simulink model "arduino_smart_plant1"  (R2024a)
settings: Solver=FixedStepAuto  StartTime=0.0  StopTime=30  RelTol=1e-3  EnableMultiTasking=on
undefined symbols (not defined in the file): Fi, Wi
libraries: arduinolib x5, arduinowifilib x4
settings Model: ExtModeTrigDuration=2  Creator=The MathWorks, Inc.  LastModifiedBy=josep
settings SolverCC: AlgebraicLoopSolver=TrustRegion
settings DataIOCC: ReturnWorkspaceOutputs=off
settings OptimizationCC: MaxStackSize=64
settings DebuggingCC: ParameterTunabilityLossMsg=error  UnconnectedInputMsg=warning  UnconnectedOutputMsg=warning  UnconnectedLineMsg=warning  ArithmeticOperatorsInVariantConditions=warning
settings HardwareCC: ProdBitPerInt=16  ProdBitPerPointer=16  ProdBitPerSizeT=16  ProdBitPerPtrDiffT=16  ProdLargestAtomicFloat=None  ProdWordSize=8  ProdHWDeviceType=Atmel->AVR  UseEmbeddedCoderFeatures=off  UseSimulinkCoderFeatures=off
settings ModelReferenceCC: EnableRefExpFcnMdlSchedulingChecks=on
settings SFSimCC: SimUseLocalCustomCode=off
settings RTWCC: Description=Embedded Coder  SystemTargetFile=ert.tlc  HardwareBoard=Arduino Mega 2560  TemplateMakefile=ert_default_tmf  GenerateReport=on  RTWUseLocalCustomCode=off  Toolchain=Arduino AVR  BuildConfiguration=Faster Runs  LaunchReport=on  GPUComputeCapability=3.5
settings CodeAppCC: ForceParamTrailComments=on  OperatorAnnotations=on  StateflowObjectComments=on  MATLABSourceComments=on
settings ERTTargetCC: ERTCustomFileBanners=off  SupportContinuousTime=on  SupportNonInlinedSFcns=on  RemoveResetFunc=off  SupportVariableSizeSignals=on  ModelStepFunctionPrototypeControlCompliant=off

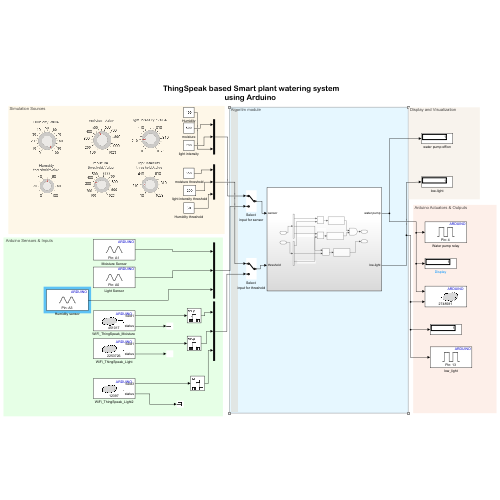
[thumbnail: Simulink's stored preview of the top-level diagram]
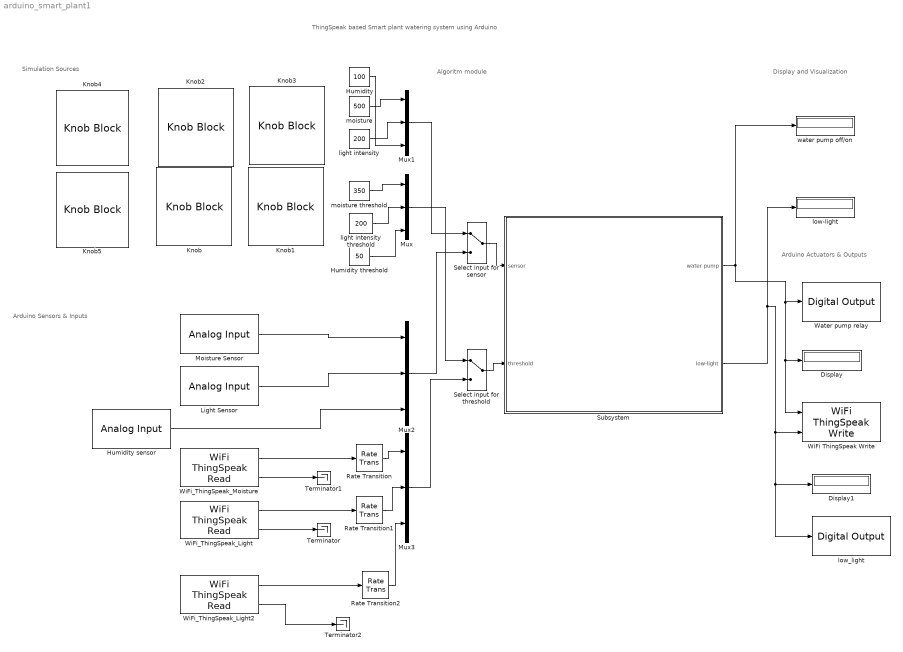
== system arduino_smart_plant1 ==
  note: Display and Visualization
  note: ThingSpeak based Smart plant watering system
      | using Arduino
  note: Simulation Sources
  note: Algoritm module
  note: Arduino Sensors & Inputs
  note: Arduino Actuators & Outputs
  " moisture threshold" : Constant  Value=350  OutDataTypeStr=uint16  SampleTime=2
  Display : Display
  Display1 : Display
  Humidity : Constant  Value=100  OutDataTypeStr=uint16
  Humidity sensor : arduinolib/Analog Input  pinNumber=3  ReadResultsOnly=off  ConversionTriggerSource=Software  ExternalTriggerType=uint32(0)  OutputDataType=uint16  EnableConversionCompleteNotify=off  EnableOuputStatus=off  SampleTime=2  blockPlatform=arduino
  Humidity threshold : Constant  Value=50  OutDataTypeStr=uint16
  Knob : KnobBlock  ScaleMin=100  ScaleMax=1023
  Knob1 : KnobBlock  ScaleMin=10  ScaleMax=1023
  Knob2 : KnobBlock  ScaleMin=100  ScaleMax=1023
  Knob3 : KnobBlock  ScaleMin=10  ScaleMax=1023
  Knob4 : KnobBlock
  Knob5 : KnobBlock
  Light Sensor : arduinolib/Analog Input  pinNumber=0  ReadResultsOnly=off  ConversionTriggerSource=Software  ExternalTriggerType=uint32(0)  OutputDataType=uint16  EnableConversionCompleteNotify=off  EnableOuputStatus=off  SampleTime=2  blockPlatform=arduino
  Moisture Sensor : arduinolib/Analog Input  pinNumber=1  ReadResultsOnly=off  ConversionTriggerSource=Software  ExternalTriggerType=uint32(0)  OutputDataType=uint16  EnableConversionCompleteNotify=off  EnableOuputStatus=off  SampleTime=2  blockPlatform=arduino
  Mux{,1..3} (4 alike) : Mux  Inputs=3
  Rate Transition : RateTransition  OutPortSampleTime=2
  Rate Transition1 : RateTransition  OutPortSampleTime=2
  Rate Transition2 : RateTransition  OutPortSampleTime=2
  Select input for sensor : ManualSwitch
  Select input for threshold : ManualSwitch
  Subsystem : Subsystem
  Terminator : Terminator
  Terminator1 : Terminator
  Terminator2 : Terminator
  Water pump relay : arduinolib/Digital Output  pinNumber=4  Direction=output  blockPlatform=arduino
  WiFi ThingSpeak Write : arduinowifilib/WiFi ThingSpeak Write  ChannelID_=2748581  WriteAPIKey_=UNYHGPLO1FA0NQNB  FieldsToWrite=[1 2]  UpdateInterval_=2  PrintDiagnosticMessages_=off  LocationEnabled=off  LocationSource=Block dialog  blockPlatform=arduino  Interfacetype_=Wi-Fi  UpdateURL=0  StatusMessage=0  StatusEnabled=on  StatusSource=<empty>
  WiFi_ThingSpeak_Light : arduinowifilib/WiFi ThingSpeak Read  ChannelID_=2253726  ChannelAccess_=Public  ReadAPIKey_=ABCDEFGHIJK  FieldsToRead_=1  PrintDiagnosticMessages_=off  blockPlatform=Arduino  Interfacetype_=Wi-Fi  SampleTime_=2
  WiFi_ThingSpeak_Light2 : arduinowifilib/WiFi ThingSpeak Read  ChannelID_=12397  ChannelAccess_=Public  ReadAPIKey_=ABCDEFGHIJK  FieldsToRead_=3  PrintDiagnosticMessages_=off  blockPlatform=Arduino  Interfacetype_=Wi-Fi  SampleTime_=60
  "WiFi_ThingSpeak_Moisture " : arduinowifilib/WiFi ThingSpeak Read  ChannelID_=451017  ChannelAccess_=Public  ReadAPIKey_=ABCDEFGHIJK  FieldsToRead_=1  PrintDiagnosticMessages_=off  blockPlatform=Arduino  Interfacetype_=Wi-Fi  SampleTime_=2
  "light intensity " : Constant  Value=200  OutDataTypeStr=uint16  SampleTime=2
  light intensity threshold : Constant  Value=200  OutDataTypeStr=uint16  SampleTime=2
  low-light : Display
  low_light : arduinolib/Digital Output  pinNumber=13  Direction=output  blockPlatform=arduino
  moisture : Constant  Value=500  OutDataTypeStr=uint16  SampleTime=2
  water pump off/on : Display
  wires:
  "light intensity "/1 -> Mux1/2
  Rate Transition/1 -> Mux3/1
  Subsystem/2(low-light) -> Display1/1, low_light/1, WiFi ThingSpeak Write/2, low-light/1
  WiFi_ThingSpeak_Light/2 -> Terminator/1
  Subsystem/1(water pump) -> water pump off/on/1, WiFi ThingSpeak Write/1, Display/1, Water pump relay/1
  "WiFi_ThingSpeak_Moisture "/1 -> Rate Transition/1
  Rate Transition1/1 -> Mux3/2
  light intensity threshold/1 -> Mux/2
  " moisture threshold"/1 -> Mux/1
  moisture/1 -> Mux1/1
  Moisture Sensor/1 -> Mux2/1
  Light Sensor/1 -> Mux2/2
  Mux1/1 -> Select input for sensor/1
  Mux2/1 -> Select input for sensor/2
  "WiFi_ThingSpeak_Moisture "/2 -> Terminator1/1
  Mux3/1 -> Select input for threshold/2
  WiFi_ThingSpeak_Light/1 -> Rate Transition1/1
  Mux/1 -> Select input for threshold/1
  Humidity threshold/1 -> Mux/3
  Humidity/1 -> Mux1/3
  Humidity sensor/1 -> Mux2/3
  WiFi_ThingSpeak_Light2/2 -> Terminator2/1
  WiFi_ThingSpeak_Light2/1 -> Rate Transition2/1
  Rate Transition2/1 -> Mux3/3
  Select input for threshold/1 -> Subsystem/2(threshold)
  Select input for sensor/1 -> Subsystem/1(sensor)

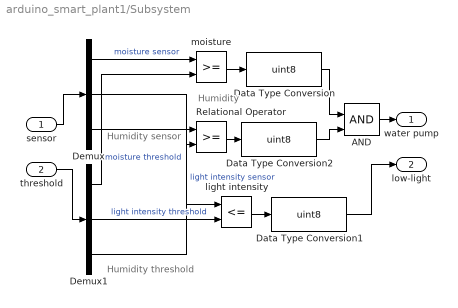
== system arduino_smart_plant1/Subsystem ==
  note: Humidity sensor
  note: Humidity threshold
  note: Humidity
  sensor : Inport
  threshold : Inport  Port=2
  AND : Logic  IconShape=distinctive  AllPortsSameDT=off  OutDataTypeStr=boolean
  Data Type Conversion : DataTypeConversion  OutDataTypeStr=uint8  SaturateOnIntegerOverflow=off  RndMeth=Floor
  Data Type Conversion1 : DataTypeConversion  OutDataTypeStr=uint8  SaturateOnIntegerOverflow=off  RndMeth=Floor
  Data Type Conversion2 : DataTypeConversion  OutDataTypeStr=uint8  SaturateOnIntegerOverflow=off  RndMeth=Floor
  Demux : Demux  Outputs=3
  Demux1 : Demux  Outputs=3
  Relational Operator : RelationalOperator  OutDataTypeStr=boolean  RndMeth=Simplest  InputSameDT=off
  "light intensity " : RelationalOperator  Operator=<=  OutDataTypeStr=boolean  RndMeth=Simplest  InputSameDT=off
  "moisture " : RelationalOperator  OutDataTypeStr=boolean  RndMeth=Simplest  InputSameDT=off
  water pump : Outport  VectorParamsAs1DForOutWhenUnconnected=off
  low-light : Outport  Port=2  VectorParamsAs1DForOutWhenUnconnected=off
  wires:
  Demux1/3 -> Relational Operator/2
  Relational Operator/1 -> Data Type Conversion2/1
  Demux1/2 -> "light intensity "/2  "light intensity threshold"
  sensor/1 -> Demux/1
  threshold/1 -> Demux1/1
  "moisture "/1 -> Data Type Conversion/1
  Demux/1 -> "moisture "/1  "moisture sensor"
  Data Type Conversion1/1 -> low-light/1
  Demux/2 -> "light intensity "/1  "light intensity sensor"
  Demux1/1 -> "moisture "/2  "moisture threshold"
  AND/1 -> water pump/1
  Data Type Conversion2/1 -> AND/2
  Demux/3 -> Relational Operator/1
  "light intensity "/1 -> Data Type Conversion1/1
  Data Type Conversion/1 -> AND/1
